simulink subsystem "Spacecraft_Dynamics"  (R2021b)
settings: Solver=VariableStepAuto  StartTime=0.0  StopTime=10.0  RelTol=1e-3
model mask{Mass=1, J=eye(3)}
  mask prompts: Mass "Mass(Kg)"; J "J(Kg*m^2)"
settings Model: Creator=DELL  LastModifiedBy=DELL

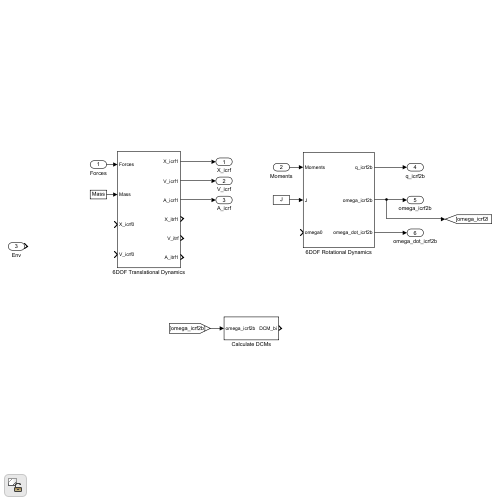
[thumbnail: Simulink's stored preview of the top-level diagram]
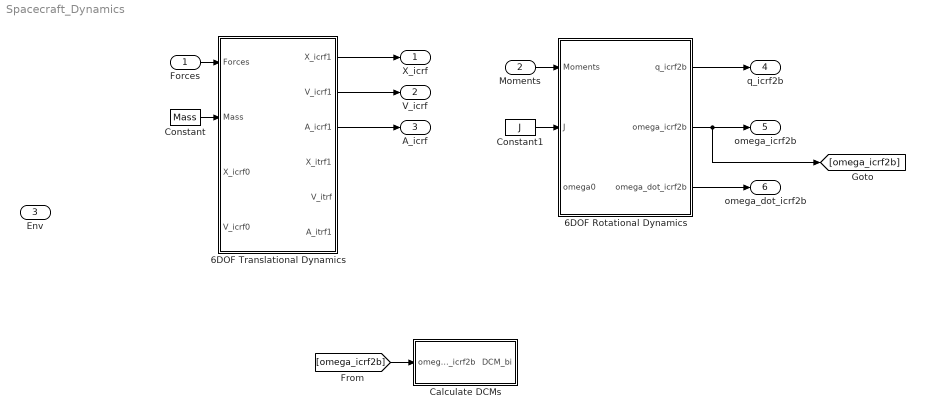
== system Spacecraft_Dynamics ==
  Forces : Inport
  Moments : Inport  Port=2
  Env : Inport  Port=3
  6DOF Rotational Dynamics : Subsystem
  6DOF Translational Dynamics : Subsystem
  Calculate DCMs : Subsystem
  Constant : Constant  Value=Mass
  Constant1 : Constant  Value=J
  X_icrf : Outport
  V_icrf : Outport  Port=2
  A_icrf : Outport  Port=3
  q_icrf2b : Outport  Port=4
  omega_icrf2b : Outport  Port=5
  omega_dot_icrf2b : Outport  Port=6
  wires:
  6DOF Translational Dynamics/1(X_icrf1) -> X_icrf/1
  6DOF Translational Dynamics/2(V_icrf1) -> V_icrf/1
  6DOF Translational Dynamics/3(A_icrf1) -> A_icrf/1
  Constant/1 -> 6DOF Translational Dynamics/2(Mass)
  Forces/1 -> 6DOF Translational Dynamics/1(Forces)
  Constant1/1 -> 6DOF Rotational Dynamics/2(J)
  Moments/1 -> 6DOF Rotational Dynamics/1(Moments)
  6DOF Rotational Dynamics/1(q_icrf2b) -> q_icrf2b/1
  6DOF Rotational Dynamics/3(omega_dot_icrf2b) -> omega_dot_icrf2b/1
  6DOF Rotational Dynamics/2(omega_icrf2b) -> omega_icrf2b/1, [omega_icrf2b]
  [omega_icrf2b] -> Calculate DCMs/1(omega_icrf2b)

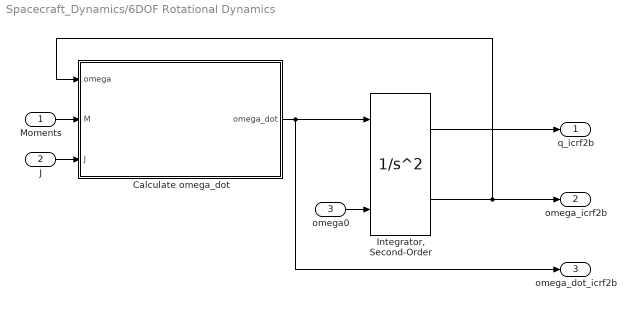
== system Spacecraft_Dynamics/6DOF Rotational Dynamics ==
  Moments : Inport
  J : Inport  Port=2
  omega0 : Inport  Port=3
  Calculate omega_dot : MATLAB Function  TreatAsAtomicUnit=on
  "Integrator, Second-Order" : SecondOrderIntegrator  ICSourceX=external  ICSourceDXDT=external
  q_icrf2b : Outport
  omega_icrf2b : Outport  Port=2
  omega_dot_icrf2b : Outport  Port=3
  wires:
  "Integrator, Second-Order"/1 -> q_icrf2b/1
  "Integrator, Second-Order"/2 -> omega_icrf2b/1, Calculate omega_dot/1(omega)
  omega0/1 -> "Integrator, Second-Order"/3
  Calculate omega_dot/1(omega_dot) -> omega_dot_icrf2b/1, "Integrator, Second-Order"/1
  J/1 -> Calculate omega_dot/3(J)
  Moments/1 -> Calculate omega_dot/2(M)

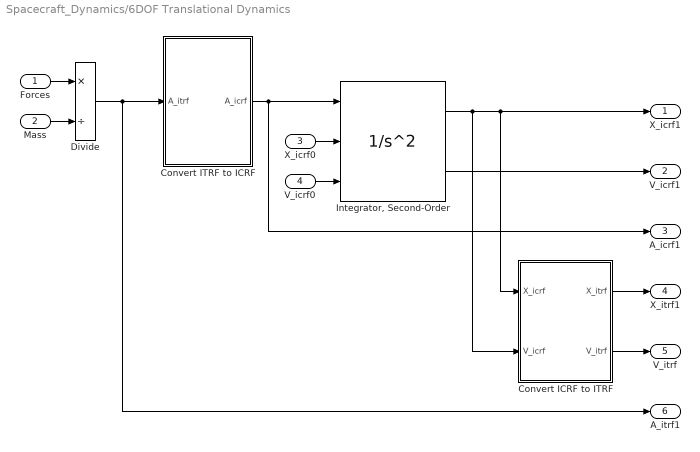
== system Spacecraft_Dynamics/6DOF Translational Dynamics ==
  Forces : Inport
  Mass : Inport  Port=2
  X_icrf0 : Inport  Port=3
  V_icrf0 : Inport  Port=4
  Convert ICRF to ITRF : MATLAB Function  TreatAsAtomicUnit=on
  Convert ITRF to ICRF : MATLAB Function  TreatAsAtomicUnit=on
  Divide : Product  Inputs=*/
  "Integrator, Second-Order" : SecondOrderIntegrator  ICSourceX=external  ICSourceDXDT=external
  X_icrf1 : Outport
  V_icrf1 : Outport  Port=2
  A_icrf1 : Outport  Port=3
  X_itrf1 : Outport  Port=4
  V_itrf : Outport  Port=5
  A_itrf1 : Outport  Port=6
  wires:
  Divide/1 -> Convert ITRF to ICRF/1(A_itrf), A_itrf1/1
  Forces/1 -> Divide/1
  Mass/1 -> Divide/2
  V_icrf0/1 -> "Integrator, Second-Order"/3
  X_icrf0/1 -> "Integrator, Second-Order"/2
  Convert ICRF to ITRF/2(V_itrf) -> V_itrf/1
  Convert ICRF to ITRF/1(X_itrf) -> X_itrf1/1
  "Integrator, Second-Order"/2 -> V_icrf1/1
  "Integrator, Second-Order"/1 -> X_icrf1/1, Convert ICRF to ITRF/1(X_icrf), Convert ICRF to ITRF/2(V_icrf)
  Convert ITRF to ICRF/1(A_icrf) -> "Integrator, Second-Order"/1, A_icrf1/1

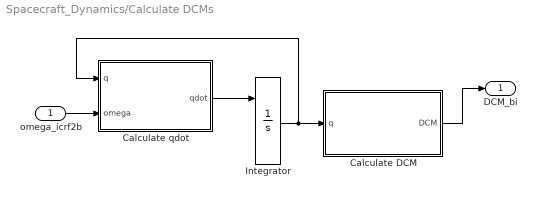
== system Spacecraft_Dynamics/Calculate DCMs ==
  omega_icrf2b : Inport
  Calculate DCM : MATLAB Function  TreatAsAtomicUnit=on
  Calculate qdot : MATLAB Function  TreatAsAtomicUnit=on
  Integrator : Integrator  InitialConditionSource=external
  DCM_bi : Outport
  wires:
  Calculate DCM/1(DCM) -> DCM_bi/1
  Integrator/1 -> Calculate DCM/1(q), Calculate qdot/1(q)
  Calculate qdot/1(qdot) -> Integrator/1
  omega_icrf2b/1 -> Calculate qdot/2(omega)

== matlab function Spacecraft_Dynamics/6DOF Translational Dynamics/Convert ITRF to ICRF ==
  data: A_itrf input; A_icrf output
function A_icrf  = fcn(A_itrf)

A_icrf = A_itrf;

== matlab function Spacecraft_Dynamics/6DOF Rotational Dynamics/Calculate omega_dot ==
  data: omega input; M input; omega_dot output; J input
function omega_dot = fcn(omega, M, J)

omega_dot = (M - omega * (J * omega)) / J;

== matlab function Spacecraft_Dynamics/Calculate DCMs/Calculate qdot ==
  data: q input; qdot output; omega input
function qdot = fcn(q, omega)

q = normalize(q);
omega_matrix = [
    0 -omega(1) -omega(2) -omega(3); 
    omega(1) 0 omega(3) -omega(2); 
    omega(2) -omega(3) 0 omega(1);
    omega(3) omega(2) -omega(1) 0];

qdot = 0.5*omega_matrix*q;

== matlab function Spacecraft_Dynamics/Calculate DCMs/Calculate DCM ==
  data: q input; DCM output
function DCM = fcn(q)
q = normalize(q);
q0 = q(1);
q1 = q(2);
q2 = q(3);
q3 = q(4);
DCM = [
    q0^2+q1^2-q2^2-q3^2 2*(q1*q2-q0*q3) 2*(q1*q3+q0*q2);
    2*(q1*q2+q0*q3) q0^2-q1^2+q2^2-q3^2 2*(q2*q3-q0*q1);
    2*(q1*q3-q0*q2) 2*(q2*q3+q0*q1) q0^2-q1^2-q2^2+q3^2;
    ];

== matlab function Spacecraft_Dynamics/6DOF Translational Dynamics/Convert ICRF to ITRF ==
  data: X_icrf input; X_itrf output; V_itrf output; V_icrf input
function [X_itrf, V_itrf] = fcn(X_icrf, V_icrf)
%#codegen

X_itrf = X_icrf;
V_itrf = V_icrf;
